simulink model "Boost_ACM"  (R2024a)
settings: Solver=VariableStepAuto  StartTime=0.0  StopTime=.2  FixedStep=1e-3  RelTol=1e-3  EnableMultiTasking=on
values from neighbouring files (symbols this model uses):
  C = 33e-6    (= 3.3e-05)    [Parameters.m]
  H = .0075    (= 0.0075)    [Parameters.m]
  L = 250e-6    (= 0.00025)    [Parameters.m]
  R = Vo^(2)/Po    (= 80)    [Parameters.m]
  Rf = .25    (= 0.25)    [Parameters.m]
  Vc = Rf*Iin    (= 2.94117647059)    [Parameters.m]
  Vin = 170    [Parameters.m]
  Vm = 4    [Parameters.m]
  Vo = 400    [Parameters.m]
settings Model: Creator=User  LastModifiedBy=User
settings OptimizationCC: DefaultParameterBehavior=Inlined  DefaultUnderspecifiedDataType=single  EnhancedBackFolding=on  PassReuseOutputArgsAs=Individual arguments  ZeroExternalMemoryAtStartup=off  MaxStackSize=64  OptimizeBlockOrder=speed  DifferentSizesBufferReuse=on  OptimizationCustomize=off  EfficientTunableParamExpr=on
settings DebuggingCC: IgnoredZcDiagnostic=none  ParameterTunabilityLossMsg=error
settings HardwareCC: ProdBitPerChar=16  ProdBitPerInt=16  ProdBitPerPointer=32  ProdBitPerSizeT=32  ProdBitPerPtrDiffT=32  ProdLargestAtomicInteger=Integer  ProdLargestAtomicFloat=None  ProdWordSize=16  ProdLongLongMode=on  ProdHWDeviceType=Texas Instruments->C2000  HardwareBoardFeatureSet=SoCBlockset
settings SFSimCC: MATLABDynamicMemAlloc=off
settings RTWCC: Description=Embedded Coder  SystemTargetFile=ert.tlc  TemplateMakefile=ert_default_tmf  Toolchain=Texas Instruments Code Composer Studio (C2000)
settings CodeAppCC: ForceParamTrailComments=on  IgnoreCustomStorageClasses=off  OperatorAnnotations=on  SimulinkDataObjDesc=on  SFDataObjDesc=on  InsertBlockDesc=on
settings ERTTargetCC: ExtModeStaticAllocSize=10000  InlinedParameterPlacement=NonHierarchical  ERTCustomFileTemplate=example_file_process.tlc

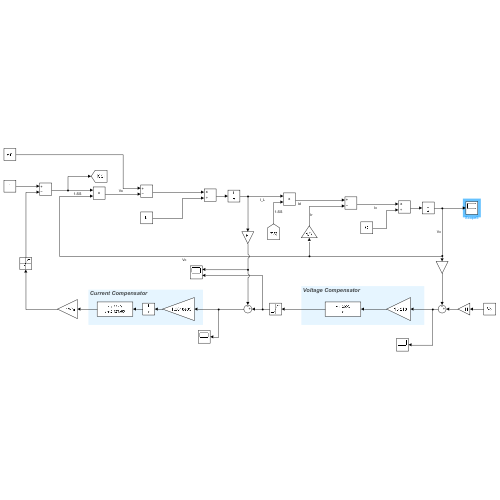
[thumbnail: Simulink's stored preview of the top-level diagram]
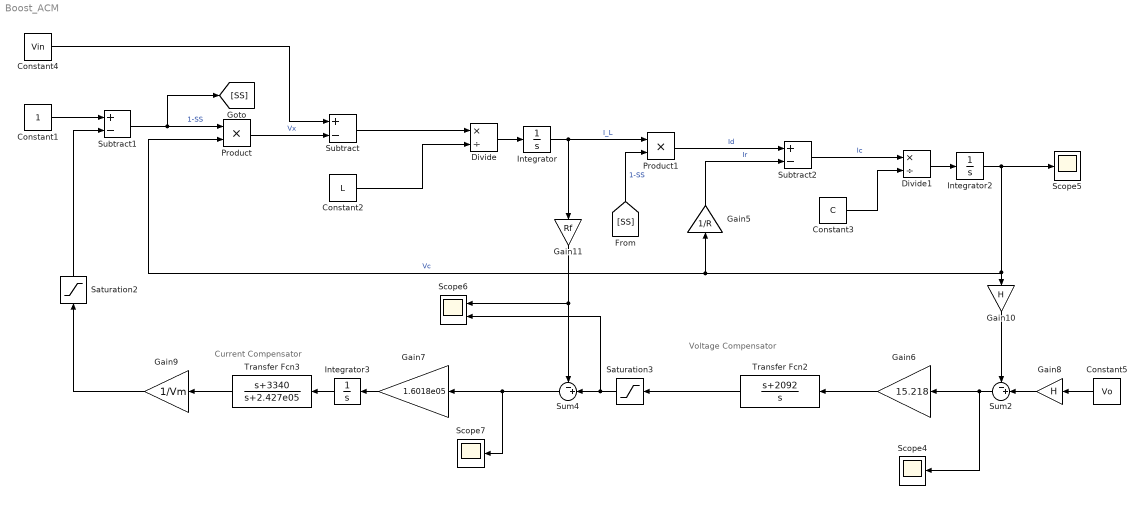
== system Boost_ACM ==
  note: Voltage Compensator
  note: Current Compensator
  Constant1 : Constant
  Constant2 : Constant  Value=L
  Constant3 : Constant  Value=C
  Constant4 : Constant  Value=Vin
  Constant5 : Constant  Value=Vo
  Divide : Product  Inputs=*/
  Divide1 : Product  Inputs=*/
  Gain10 : Gain  Gain=H
  Gain11 : Gain  Gain=Rf
  Gain5 : Gain  Gain=1/R
  Gain6 : Gain  Gain=15.218
  Gain7 : Gain  Gain=1.6018e05
  Gain8 : Gain  Gain=H
  Gain9 : Gain  Gain=1/Vm
  Integrator : Integrator  LowerSaturationLimit=0
  Integrator2 : Integrator  LowerSaturationLimit=0
  Integrator3 : Integrator
  Product : Product
  Product1 : Product
  Saturation2 : Saturate  UpperLimit=.9  LowerLimit=.1
  Saturation3 : Saturate  UpperLimit=Vc  LowerLimit=0
  Scope4 : Scope
  Scope5 : Scope
  Scope6 : Scope  NumInputPorts=2
  Scope7 : Scope
  Subtract : Sum  Inputs=+-
  Subtract1 : Sum  Inputs=+-
  Subtract2 : Sum  Inputs=+-
  Sum2 : Sum  Inputs=-+|
  Sum4 : Sum  Inputs=-+|
  Transfer Fcn2 : TransferFcn  Numerator=[1 2092]  Denominator=[1 0]
  Transfer Fcn3 : TransferFcn  Numerator=[1 3340]  Denominator=[1 2.427e05]
  wires:
  Integrator2/1 -> Scope5/1, Gain5/1, Product/2, Gain10/1  "Vc"
  Constant2/1 -> Divide/2
  Divide/1 -> Integrator/1
  Integrator/1 -> Product1/1, Gain11/1  "I_L"
  Product1/1 -> Subtract2/1  "Id"
  Subtract2/1 -> Divide1/1  "Ic"
  Gain5/1 -> Subtract2/2  "Ir"
  Subtract1/1 -> [SS], Product/1  "1-SS"
  [SS] -> Product1/2  "1-SS"
  Divide1/1 -> Integrator2/1
  Subtract/1 -> Divide/1
  Constant3/1 -> Divide1/2
  Constant4/1 -> Subtract/1
  Gain9/1 -> Saturation2/1
  Product/1 -> Subtract/2  "Vx"
  Constant1/1 -> Subtract1/1
  Gain8/1 -> Sum2/2
  Transfer Fcn2/1 -> Saturation3/1
  Gain10/1 -> Sum2/1
  Integrator3/1 -> Transfer Fcn3/1
  Gain7/1 -> Integrator3/1
  Sum4/1 -> Scope7/1, Gain7/1
  Gain6/1 -> Transfer Fcn2/1
  Sum2/1 -> Gain6/1, Scope4/1
  Constant5/1 -> Gain8/1
  Transfer Fcn3/1 -> Gain9/1
  Gain11/1 -> Sum4/1, Scope6/1
  Saturation2/1 -> Subtract1/2
  Saturation3/1 -> Scope6/2, Sum4/2
